simulink model "servo"  (R2024a)
settings: Solver=VariableStepAuto  StartTime=0.0  StopTime=50.0  RelTol=1e-3
undefined symbols (not defined in the file): a, b, Beta, Bm, Jm, K, Ka, Kb, La, Ra
settings Model: Creator=Ricky  LastModifiedBy=Ricky

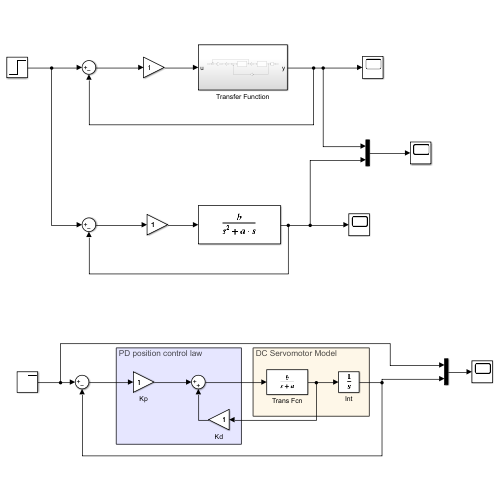
[thumbnail: Simulink's stored preview of the top-level diagram]
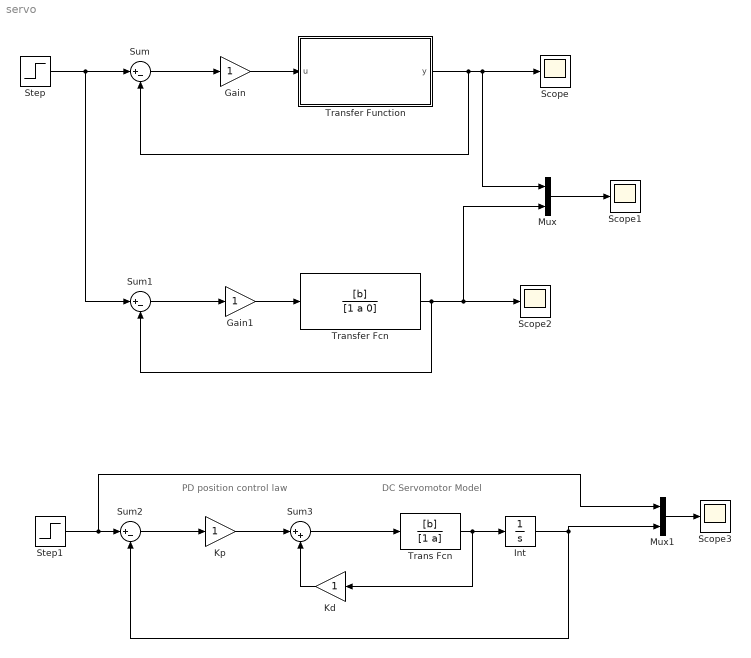
== system servo ==
  note: DC Servomotor Model
  note: PD position control law
  Gain : Gain
  Gain1 : Gain
  Int : Integrator
  Kd : Gain
  Kp : Gain
  Mux : Mux  Inputs=2
  Mux1 : Mux  Inputs=2
  Scope{,1..3} (4 alike) : Scope
  Step : Step  SampleTime=0
  Step1 : Step  SampleTime=0
  Sum : Sum  Inputs=|+-
  Sum1 : Sum  Inputs=|+-
  Sum2 : Sum  Inputs=|+-
  Sum3 : Sum  Inputs=|++
  Trans Fcn : TransferFcn  Numerator=[b]  Denominator=[1 a]
  Transfer Fcn : TransferFcn  Numerator=[b]  Denominator=[1 a 0]
  Transfer Function : Subsystem
  wires:
  Gain/1 -> Transfer Function/1(u)
  Sum/1 -> Gain/1
  Step/1 -> Sum1/1, Sum/1
  Transfer Function/1(y) -> Sum/2, Mux/1, Scope/1
  Mux/1 -> Scope1/1
  Transfer Fcn/1 -> Sum1/2, Mux/2, Scope2/1
  Gain1/1 -> Transfer Fcn/1
  Sum1/1 -> Gain1/1
  Step1/1 -> Mux1/1, Sum2/1
  Sum2/1 -> Kp/1
  Kp/1 -> Sum3/1
  Trans Fcn/1 -> Kd/1, Int/1
  Sum3/1 -> Trans Fcn/1
  Mux1/1 -> Scope3/1
  Int/1 -> Mux1/2, Sum2/2
  Kd/1 -> Sum3/2

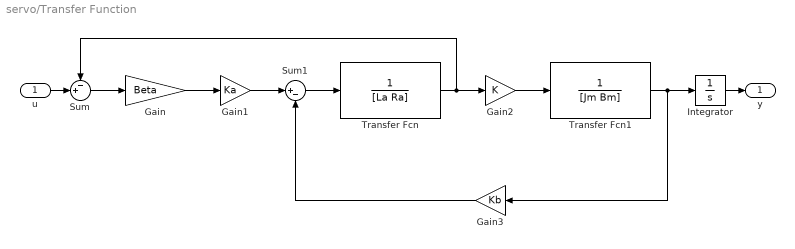
== system servo/Transfer Function ==
  u : Inport
  Gain : Gain  Gain=Beta
  Gain1 : Gain  Gain=Ka
  Gain2 : Gain  Gain=K
  Gain3 : Gain  Gain=Kb
  Integrator : Integrator
  Sum : Sum  Inputs=-+|
  Sum1 : Sum  Inputs=|+-
  Transfer Fcn : TransferFcn  Denominator=[La Ra]
  Transfer Fcn1 : TransferFcn  Denominator=[Jm Bm]
  y : Outport
  wires:
  Transfer Fcn1/1 -> Gain3/1, Integrator/1
  Sum1/1 -> Transfer Fcn/1
  Gain/1 -> Gain1/1
  Integrator/1 -> y/1
  Gain1/1 -> Sum1/1
  Transfer Fcn/1 -> Sum/1, Gain2/1
  Gain3/1 -> Sum1/2
  Gain2/1 -> Transfer Fcn1/1
  Sum/1 -> Gain/1
  u/1 -> Sum/2
